simulink subsystem "Sennalizador"  (R2023b)
settings: Solver=VariableStepAuto  StartTime=0.0  StopTime=10.0  RelTol=1e-3
libraries: simulink x8
settings Model: Creator=johan  LastModifiedBy=johan

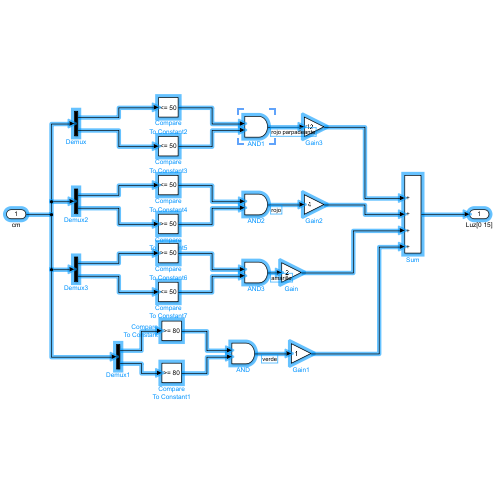
[thumbnail: Simulink's stored preview of the top-level diagram]
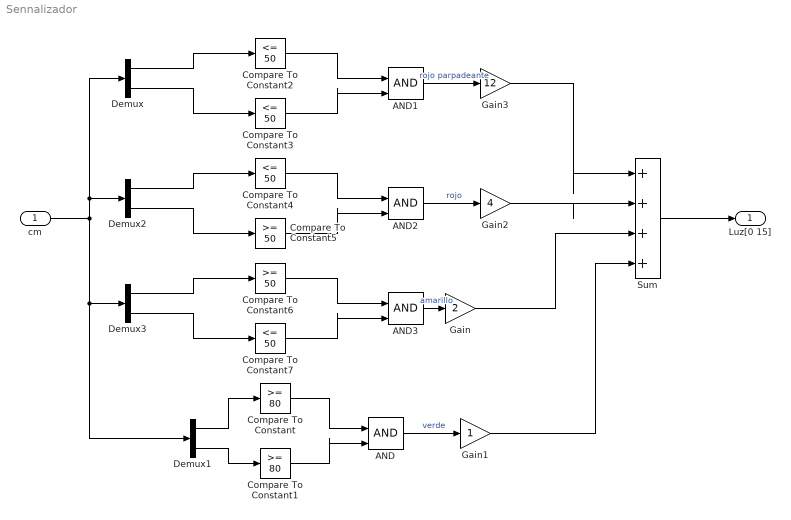
== system Sennalizador ==
  cm : Inport
  AND{,1..3} (4 alike) : Logic  IconShape=distinctive  AllPortsSameDT=off  OutDataTypeStr=boolean
  Compare To Constant : simulink/Logic and Bit Operations/Compare To Constant  relop=>=  const=80  OutDataTypeStr=boolean
  Compare To Constant1 : simulink/Logic and Bit Operations/Compare To Constant  relop=>=  const=80  OutDataTypeStr=boolean
  Compare To Constant{2..4,7} (4 alike) : simulink/Logic and Bit Operations/Compare To Constant  relop=<=  const=50  OutDataTypeStr=boolean
  Compare To Constant5 : simulink/Logic and Bit Operations/Compare To Constant  relop=>=  const=50  OutDataTypeStr=boolean
  Compare To Constant6 : simulink/Logic and Bit Operations/Compare To Constant  relop=>=  const=50  OutDataTypeStr=boolean
  Demux{,1..3} (4 alike) : Demux  Outputs=2
  Gain : Gain  Gain=2
  Gain1 : Gain
  Gain2 : Gain  Gain=4
  Gain3 : Gain  Gain=12
  Sum : Sum  Inputs=|++++
  Luz[0 15] : Outport
  wires:
  Demux1/2 -> Compare To Constant1/1
  Gain2/1 -> Sum/2
  Compare To Constant1/1 -> AND/2
  Gain1/1 -> Sum/4
  Demux/2 -> Compare To Constant3/1
  Demux/1 -> Compare To Constant2/1
  Compare To Constant7/1 -> AND3/2
  cm/1 -> Demux3/1, Demux1/1, Demux2/1, Demux/1
  Demux3/1 -> Compare To Constant6/1
  AND/1 -> Gain1/1  "verde"
  Compare To Constant3/1 -> AND1/2
  Compare To Constant2/1 -> AND1/1
  Demux3/2 -> Compare To Constant7/1
  Compare To Constant4/1 -> AND2/1
  Compare To Constant5/1 -> AND2/2
  Sum/1 -> Luz[0 15]/1
  Demux2/2 -> Compare To Constant5/1
  AND1/1 -> Gain3/1  "rojo parpadeante"
  AND2/1 -> Gain2/1  "rojo"
  Compare To Constant/1 -> AND/1
  Demux2/1 -> Compare To Constant4/1
  Gain/1 -> Sum/3
  Demux1/1 -> Compare To Constant/1
  Gain3/1 -> Sum/1
  Compare To Constant6/1 -> AND3/1
  AND3/1 -> Gain/1  "amarillo"
